simulink model "IBC_open_basis_test_SMC_False"  (R2019b)
settings: Solver=VariableStepAuto  StartTime=0.0  StopTime=0.03  RelTol=1e-3
InitFcn:
  | Load=2;
  | C=370e-6;
  | L1=1000e-6;
  | L2=1000e-6*(1+normrnd(0,0.05,[1,1]));
  | L3=1000e-6*(1+normrnd(0,0.05,[1,1]));
  | alp=1-0.5;
  | V = 12;
  | L = 1000e-6;
  | D = 0.5;
  | Vg= 12;
  | R = 2;
libraries: powerlib x25, dspsigops x3, powerlib_meascontrol x2
settings Model: SimulationMode=accelerator  Creator=mahdi  LastModifiedBy=29721
settings DataIOCC: ReturnWorkspaceOutputs=off
settings DebuggingCC: ArithmeticOperatorsInVariantConditions=warning
settings SFSimCC: SimUseLocalCustomCode=off  CustomCodeUndefinedFunction=UseInterfaceOnly
settings RTWCC: RTWUseLocalCustomCode=off
settings CodeAppCC: StateflowObjectComments=on
settings SimscapeCC: SimscapeNormalizeSystem=off

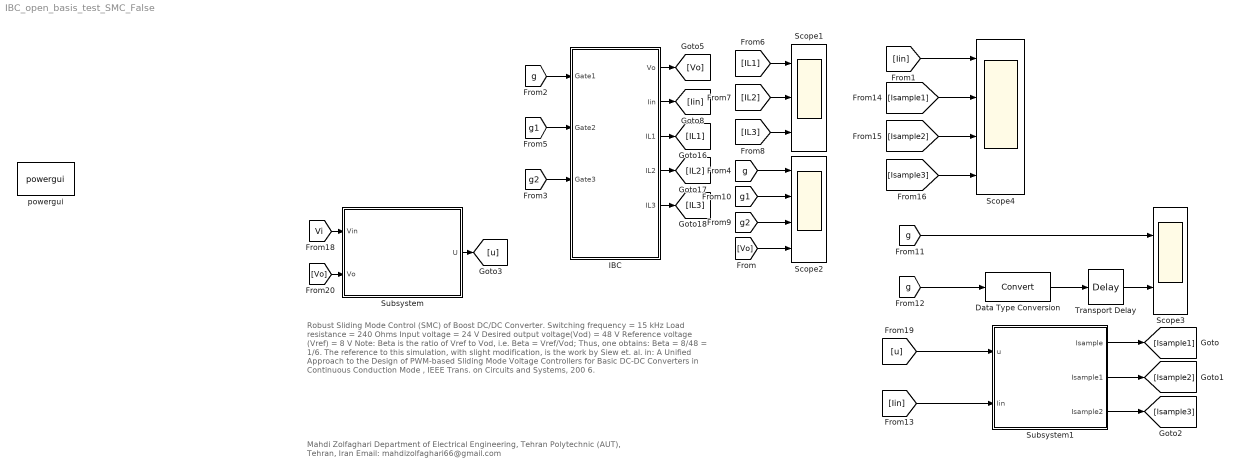
== system IBC_open_basis_test_SMC_False ==
  note: Mahdi Zolfaghari
      | Department of Electrical Engineering, Tehran Polytechnic (AUT), Tehran, Iran
      | Email: mahdizolfaghari66@gmail.com
  note: Robust Sliding Mode Control (SMC) of Boost DC/DC Converter.
      | Switching frequency = 15 kHz
      | Load resistance = 240 Ohms
      | Input voltage = 24 V
      | Desired output voltage(Vod) = 48 V
      | Reference voltage (Vref) = 8 V
      | Note: Beta is the ratio of Vref to Vod, i.e. Beta = Vref/Vod; Thus, one obtains:
      | Beta = 8/48 = 1/6.
      | The reference to this simulation, with slight modification, is the work by Siew et. al. in:
      | A Unified Approach to the Design of PWM-based Sliding Mode Voltage Controllers
      | for Basic DC-DC Converters in Continuous Conduction Mode , IEEE Trans. on Circuits and Systems, 200 6.
  Data Type Conversion : DataTypeConversion
  IBC : Subsystem  mask{L1=L1, L2=L1, L3=L1, C=C, R=R, Vin=Vg}
  Scope1 : Scope  NumInputPorts=3
  Scope2 : Scope  NumInputPorts=4
  Scope3 : Scope  NumInputPorts=2
  Scope4 : Scope  NumInputPorts=4
  Subsystem : Subsystem
      mask Display: disp('Sliding Mode\nController')
  Subsystem1 : Subsystem
  Transport Delay : TransportDelay  DelayTime=0.5*1/(15e3)/2
  powergui : powerlib/powergui  Priority=1  SimulationMode=Discrete  SampleTime=2.5e-8  frequency=60  Iterations=50  frequencyindice=0  Pbase=100e6  ErrMax=1e-4  UnitsV=kV  UnitsW=MW  buscounter=0  FunctionMessages=off  echomessages=off  EnableUseOfTLC=off  CurrentSourceSwitches=off  DisableSnubberDevices=off  DisableRonSwitches=off  DisableVfSwitches=off  DisplayEquations=off  AutomaticDiscreteSolvers=off  SolverType=Tustin/Backward Euler (TBE)  Interpol=off  ExternalGateDelay=off  methode=off  Ts=10  x0status=blocks  SPID=off  SwTol=0  HookPort=off  NonlinearTolerance=1e-4  nMaxIteration=100  ContinueOnMaxIteration=off  RestoreLinks=warning  ResistiveCurrentMeasurement=off  Frange=[0:2:500]  Ylog=off  Xlog=on  ShowGrid=off  save=off  variable=ZData  structure=0  ZoomFFT=off  StartTime=0.0  cycles=1  DisplayStyle=1  fundamental=60  FreqAxis=off  MaxFrequency=1000  frequencyindicesteady=1  RmsSteady=1  display=off
      settings: SourceProductName=Simscape Electrical
  wires:
  [g2] -> IBC/3(Gate3)
  IBC/3(IL1) -> [IL1]
  IBC/5(IL3) -> [IL3]
  [g1] -> IBC/2(Gate2)
  IBC/2(Iin) -> [Iin]
  IBC/4(IL2) -> [IL2]
  IBC/1(Vo) -> [Vo]
  [g] -> IBC/1(Gate1)
  [IL1] -> Scope1/1
  [IL3] -> Scope1/3
  [IL2] -> Scope1/2
  [g] -> Scope2/1
  [g1] -> Scope2/2
  [g2] -> Scope2/3
  [Vo] -> Scope2/4
  [g] -> Data Type Conversion/1
  [g] -> Scope3/1
  Transport Delay/1 -> Scope3/2
  Data Type Conversion/1 -> Transport Delay/1
  [u] -> Subsystem1/1(u)
  [Iin] -> Subsystem1/2(Iin)
  [Isample1] -> Scope4/2
  [Isample2] -> Scope4/3
  [Isample3] -> Scope4/4
  Subsystem1/1(Isample) -> [Isample1]
  Subsystem1/2(Isample1) -> [Isample2]
  Subsystem1/3(Isample2) -> [Isample3]
  Subsystem/1(U) -> [u]
  [Vo] -> Subsystem/2(Vo)
  [Vi] -> Subsystem/1(Vin)
  [Iin] -> Scope4/1

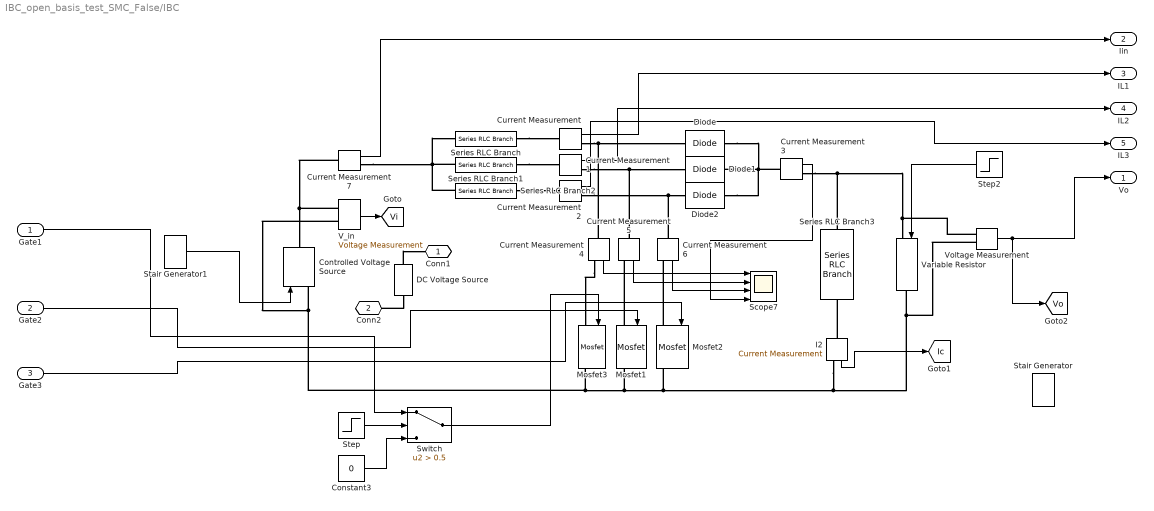
== system IBC_open_basis_test_SMC_False/IBC ==
  Gate1 : Inport
  Gate2 : Inport  Port=2
  Gate3 : Inport  Port=3
  Constant3 : Constant  Value=0
  Controlled Voltage Source : powerlib/Electrical Sources/Controlled Voltage Source  Initialize=on  Source_Type=AC  Amplitude=0  Phase=0  Frequency=0  Measurements=None
      settings: SourceProductName=Simscape Electrical
  Current Measurement{,1..7} (8 alike) : powerlib/Measurements/Current Measurement  PhasorSimulation=off  OutputType=Complex  PSBequivalent=0
      settings: SourceProductName=Simscape Electrical
  DC Voltage Source : powerlib/Electrical Sources/DC Voltage Source  Amplitude=V  Measurements=None
      settings: SourceProductName=Simscape Electrical
  Diode : powerlib/Power Electronics/Diode  Ron=0.001  Lon=0  Vf=0  IC=0  UseSnubber=0  Rs=inf  Cs=250e-9  Measurements=off
      settings: SourceProductName=Simscape Electrical
  Diode1 : powerlib/Power Electronics/Diode  Ron=0.001  Lon=0  Vf=0  IC=0  UseSnubber=0  Rs=inf  Cs=250e-9  Measurements=off
      settings: SourceProductName=Simscape Electrical
  Diode2 : powerlib/Power Electronics/Diode  Ron=0.001  Lon=0  Vf=0  IC=0  UseSnubber=0  Rs=inf  Cs=250e-9  Measurements=off
      settings: SourceProductName=Simscape Electrical
  I2 : powerlib/Measurements/Current Measurement  PhasorSimulation=off  OutputType=Complex  PSBequivalent=0
      settings: SourceProductName=Simscape Electrical
  Mosfet1 : powerlib/Power Electronics/Mosfet  Ron=0.1  Lon=0  Rd=0.01  Vfd=0  IC=0  Rs=1e5  Cs=inf  Measurements=on
      settings: SourceProductName=Simscape Electrical
  Mosfet2 : powerlib/Power Electronics/Mosfet  Ron=0.1  Lon=0  Rd=0.01  Vfd=0  IC=0  Rs=1e5  Cs=inf  Measurements=on
      settings: SourceProductName=Simscape Electrical
  Mosfet3 : powerlib/Power Electronics/Mosfet  Ron=0.1  Lon=0  Rd=0.01  Vfd=0  IC=0  Rs=1e5  Cs=inf  Measurements=on
      settings: SourceProductName=Simscape Electrical
  Scope7 : Scope  NumInputPorts=4
  Series RLC Branch : powerlib/Elements/Series RLC Branch  LConnTagsString=__new0  RConnTagsString=__new0  BranchType=RL  Resistance=0.14  Inductance=L1  SetiL0=off  InitialCurrent=0  Capacitance=1e-6  Setx0=off  InitialVoltage=0  Measurements=None
      settings: SourceProductName=Simscape Electrical
  Series RLC Branch1 : powerlib/Elements/Series RLC Branch  LConnTagsString=__new0  RConnTagsString=__new0  BranchType=RL  Resistance=0.14  Inductance=L2  SetiL0=off  InitialCurrent=0  Capacitance=1e-6  Setx0=off  InitialVoltage=0  Measurements=None
      settings: SourceProductName=Simscape Electrical
  Series RLC Branch2 : powerlib/Elements/Series RLC Branch  LConnTagsString=__new0  RConnTagsString=__new0  BranchType=RL  Resistance=0.14  Inductance=L3  SetiL0=off  InitialCurrent=0  Capacitance=1e-6  Setx0=off  InitialVoltage=0  Measurements=None
      settings: SourceProductName=Simscape Electrical
  Series RLC Branch3 : powerlib/Elements/Series RLC Branch  LConnTagsString=__new0  RConnTagsString=__new0  BranchType=RC  Resistance=0  Inductance=1e-3  SetiL0=off  InitialCurrent=0  Capacitance=C  Setx0=off  InitialVoltage=0  Measurements=None
      settings: SourceProductName=Simscape Electrical
  Stair Generator : powerlib_meascontrol/Pulse & Signal Generators/Stair Generator  t=[0,0.01,0.02]  e=[2,4,8]  Ts=0
      settings: SourceProductName=Simscape Electrical
  Stair Generator1 : powerlib_meascontrol/Pulse & Signal Generators/Stair Generator  t=[0,0.01,0.02]  e=[12,12,12]  Ts=0
      settings: SourceProductName=Simscape Electrical
  Step : Step  Time=0.02499  Before=1  After=0  SampleTime=0
  Step2 : Step  Time=0.01  Before=4  After=6  SampleTime=0
  Switch : Switch  Criteria=u2 > Threshold  Threshold=0.5
  V_in : powerlib/Measurements/Voltage Measurement  PhasorSimulation=off  OutputType=Complex  PSBequivalent=0
      settings: SourceProductName=Simscape Electrical
  Variable Resistor : powerlib/Elements/Variable Resistor  Rabsmin=1e-3
      settings: SourceProductName=Simscape Electrical  SourceProductBaseCode=PS
  Voltage Measurement : powerlib/Measurements/Voltage Measurement  PhasorSimulation=off  OutputType=Complex  PSBequivalent=0
      settings: SourceProductName=Simscape Electrical
  Conn1 : PMIOPort  Side=Right
  Conn2 : PMIOPort  Port=2  Side=Left
  Vo : Outport
  Iin : Outport  Port=2
  IL1 : Outport  Port=3
  IL2 : Outport  Port=4
  IL3 : Outport  Port=5
  tag scope: Ic=global, Vi=global, Vo=global
  wires:
  Step2/1 -> Variable Resistor/1
  Current Measurement6/1 -> Scope7/3
  Current Measurement5/1 -> Scope7/2
  Current Measurement1/1 -> IL2/1
  Current Measurement4/1 -> Scope7/1
  Current Measurement2/1 -> IL3/1
  Step/1 -> Switch/2
  Switch/1 -> Mosfet3/1
  Current Measurement3/1 -> Scope7/4
  Stair Generator1/1 -> Controlled Voltage Source/1
  Gate3/1 -> Mosfet2/1
  Voltage Measurement/1 -> [Vo], Vo/1
  Current Measurement/1 -> IL1/1
  Constant3/1 -> Switch/3
  Current Measurement7/1 -> Iin/1
  Gate1/1 -> Switch/1
  Gate2/1 -> Mosfet1/1
  V_in/1 -> [Vi]
  I2/1 -> [Ic]
  connections:
  Series RLC Branch2/RConn1 -- Current Measurement2/LConn1
  Mosfet2/LConn1 -- Current Measurement6/RConn1
  Current Measurement7/LConn1 -- V_in/LConn1 -- Controlled Voltage Source/RConn1
  Series RLC Branch/RConn1 -- Current Measurement/LConn1
  Series RLC Branch1/RConn1 -- Current Measurement1/LConn1
  Mosfet3/RConn1 -- V_in/LConn2 -- Controlled Voltage Source/LConn1 -- Mosfet1/RConn1 -- Mosfet2/RConn1 -- I2/RConn1 -- Voltage Measurement/LConn2 -- Variable Resistor/RConn1
  Mosfet1/LConn1 -- Current Measurement5/RConn1
  Current Measurement2/RConn1 -- Current Measurement6/LConn1 -- Diode2/LConn1
  DC Voltage Source/LConn1 -- Conn2/RConn1
  Current Measurement3/RConn1 -- Series RLC Branch3/LConn1 -- Voltage Measurement/LConn1 -- Variable Resistor/LConn1
  Current Measurement4/RConn1 -- Mosfet3/LConn1
  Current Measurement7/RConn1 -- Series RLC Branch2/LConn1 -- Series RLC Branch1/LConn1 -- Series RLC Branch/LConn1
  Current Measurement1/RConn1 -- Diode1/LConn1 -- Current Measurement5/LConn1
  Current Measurement3/LConn1 -- Diode2/RConn1 -- Diode/RConn1 -- Diode1/RConn1
  Current Measurement/RConn1 -- Diode/LConn1 -- Current Measurement4/LConn1
  DC Voltage Source/RConn1 -- Conn1/RConn1
  I2/LConn1 -- Series RLC Branch3/RConn1

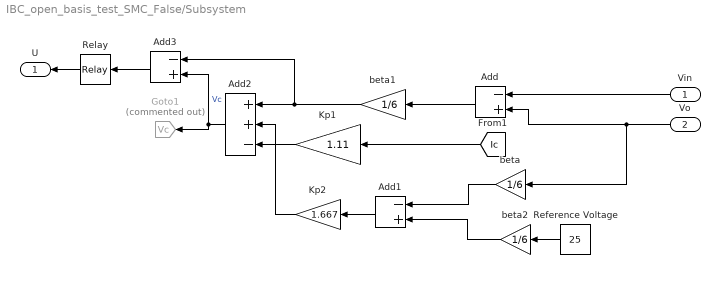
== system IBC_open_basis_test_SMC_False/Subsystem ==
  Vin : Inport
  Vo : Inport  Port=2
  Add : Sum  Inputs=-+
  Add1 : Sum  Inputs=-+
  Add2 : Sum  Inputs=++-
  Add3 : Sum  Inputs=-+
  Goto1 : Goto  Commented=on  GotoTag=Vc  TagVisibility=global
  Kp1 : Gain  Gain=1.11
  Kp2 : Gain  Gain=1.667
  Reference Voltage : Constant  Value=25
  Relay : Relay  OnSwitchValue=3.75e-3  OffSwitchValue=3.5e-3
  beta : Gain  Gain=1/6
  beta1 : Gain  Gain=1/6
  beta2 : Gain  Gain=1/6
  U : Outport
  wires:
  Add1/1 -> Kp2/1
  Add/1 -> beta1/1
  Vin/1 -> Add/1
  Kp2/1 -> Add2/2
  Add3/1 -> Relay/1
  Add2/1 -> Goto1/1, Add3/2  "Vc"
  Reference Voltage/1 -> beta2/1
  beta/1 -> Add1/1
  Kp1/1 -> Add2/3
  [Ic] -> Kp1/1
  beta1/1 -> Add3/1, Add2/1
  Vo/1 -> beta/1, Add/2
  beta2/1 -> Add1/2
  Relay/1 -> U/1

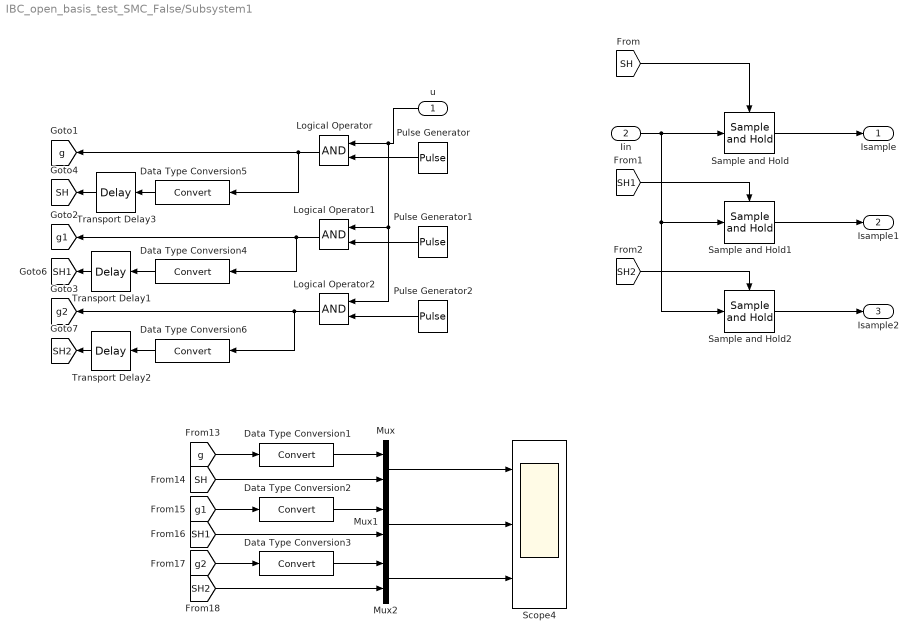
== system IBC_open_basis_test_SMC_False/Subsystem1 ==
  u : Inport
  Iin : Inport  Port=2
  Data Type Conversion{1..6} (6 alike) : DataTypeConversion
  Logical Operator : Logic  AllPortsSameDT=off  OutDataTypeStr=boolean
  Logical Operator1 : Logic  AllPortsSameDT=off  OutDataTypeStr=boolean
  Logical Operator2 : Logic  AllPortsSameDT=off  OutDataTypeStr=boolean
  Mux : Mux  Inputs=2
  Mux1 : Mux  Inputs=2
  Mux2 : Mux  Inputs=2
  Pulse Generator : DiscretePulseGenerator  PulseType=Time based  Period=1/15e3  PulseWidth=50
  Pulse Generator1 : DiscretePulseGenerator  PulseType=Time based  Period=1/15e3  PulseWidth=50  PhaseDelay=-1/15e3/3
  Pulse Generator2 : DiscretePulseGenerator  PulseType=Time based  Period=1/15e3  PulseWidth=50  PhaseDelay=1/15e3/3
  Sample and Hold : dspsigops/Sample and Hold  trig=Rising edge  initCond=0  latchinput=off
  Sample and Hold1 : dspsigops/Sample and Hold  trig=Rising edge  initCond=0  latchinput=off
  Sample and Hold2 : dspsigops/Sample and Hold  trig=Rising edge  initCond=0  latchinput=off
  Scope4 : Scope  NumInputPorts=3
  Transport Delay1 : TransportDelay  DelayTime=0.5*1/(15e3)/2
  Transport Delay2 : TransportDelay  DelayTime=0.5*1/(15e3)/2
  Transport Delay3 : TransportDelay  DelayTime=0.5*1/(15e3)/2
  Isample : Outport
  Isample1 : Outport  Port=2
  Isample2 : Outport  Port=3
  tag scope: SH1=global, SH2=global, SH=global, g1=global, g2=global, g=global
  wires:
  Data Type Conversion2/1 -> Mux1/1
  Logical Operator/1 -> Data Type Conversion5/1, [g]
  Pulse Generator/1 -> Logical Operator/2
  Pulse Generator1/1 -> Logical Operator1/2
  Pulse Generator2/1 -> Logical Operator2/2
  Mux/1 -> Scope4/1
  [g1] -> Data Type Conversion2/1
  Data Type Conversion1/1 -> Mux/1
  u/1 -> Logical Operator2/1, Logical Operator1/1, Logical Operator/1
  [SH] -> Mux/2
  Mux2/1 -> Scope4/3
  [SH2] -> Mux2/2
  [g] -> Data Type Conversion1/1
  Data Type Conversion3/1 -> Mux2/1
  [g2] -> Data Type Conversion3/1
  [SH1] -> Mux1/2
  Logical Operator1/1 -> Data Type Conversion4/1, [g1]
  Logical Operator2/1 -> Data Type Conversion6/1, [g2]
  Mux1/1 -> Scope4/2
  Transport Delay1/1 -> [SH1]
  Data Type Conversion4/1 -> Transport Delay1/1
  Data Type Conversion5/1 -> Transport Delay3/1
  Data Type Conversion6/1 -> Transport Delay2/1
  Transport Delay2/1 -> [SH2]
  Transport Delay3/1 -> [SH]
  [SH] -> Sample and Hold/Trigger
  [SH1] -> Sample and Hold1/Trigger
  [SH2] -> Sample and Hold2/Trigger
  Iin/1 -> Sample and Hold2/1, Sample and Hold1/1, Sample and Hold/1
  Sample and Hold/1 -> Isample/1
  Sample and Hold1/1 -> Isample1/1
  Sample and Hold2/1 -> Isample2/1
